simulink model "foc_pmsm"  (R2023a)
settings: Solver=VariableStepAuto  StartTime=0.0  StopTime=0.2  RelTol=1e-3
values from neighbouring files (symbols this model uses):
  L_d = 0.00113    [pmsm_init.m]    (also in pmsm_operating_points.m; pmsm_validation_compare.m)
  L_q = 0.00142    [pmsm_init.m]    (also in pmsm_operating_points.m; pmsm_validation_compare.m)
  polepairs = 3    [pmsm_init.m]    (also in pmsm_operating_points.m; pmsm_validation_compare.m)
  Psi_PM = 0.0169    [pmsm_init.m]    (also in pmsm_operating_points.m; pmsm_validation_compare.m)
  R_s = 0.543    [pmsm_init.m]    (also in pmsm_operating_points.m; pmsm_validation_compare.m)
  Ts = 1/10000    (= 0.0001)    [pmsm_init.m]    (also in pmsm_operating_points.m; pmsm_validation_compare.m)
  V_max = V_DC * max_modulation_index    [pmsm_init.m]    (also in pmsm_operating_points.m; pmsm_validation_compare.m)
undefined symbols (not defined in the file or in its folder): K_Id, K_Iq, K_Pd, K_Pq
libraries: slpidlib x2
settings Model: Creator=brogh  LastModifiedBy=hufnagelde
settings DataIOCC: SaveFormat=StructureWithTime
settings OptimizationCC: ReuseModelBlockBuffer=off
settings DebuggingCC: UnconnectedInputMsg=warning  UnconnectedOutputMsg=warning  UnconnectedLineMsg=warning
settings ModelReferenceCC: EnableRefExpFcnMdlSchedulingChecks=on
settings RTWCC: DLArmComputeVersion=19.05

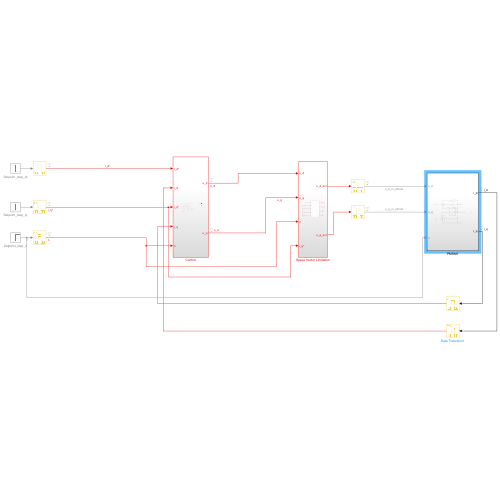
[thumbnail: Simulink's stored preview of the top-level diagram]
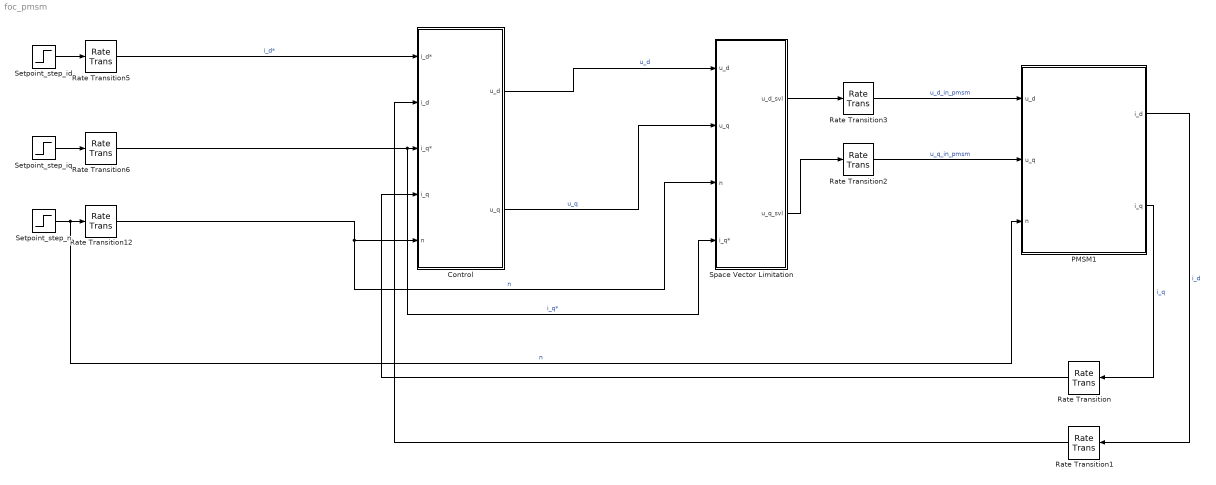
== system foc_pmsm ==
  Control : Subsystem
  PMSM1 : Subsystem
  Rate Transition{,1,5..6,12} (5 alike) : RateTransition  OutPortSampleTime=Ts
  Rate Transition2 : RateTransition  OutPortSampleTime=0
  Rate Transition3 : RateTransition  OutPortSampleTime=0
  Setpoint_step_id : Step  Time=0.1  After=-5  SampleTime=0
  Setpoint_step_iq : Step  Time=0.1  After=5  SampleTime=0
  Setpoint_step_n : Step  Time=0.03  Before=1000  After=1000  SampleTime=0
  Space Vector Limitation : Subsystem
  wires:
  Setpoint_step_id/1 -> Rate Transition5/1
  PMSM1/2(i_q) -> Rate Transition/1  "i_q"
  PMSM1/1(i_d) -> Rate Transition1/1  "i_d"
  Setpoint_step_iq/1 -> Rate Transition6/1
  Rate Transition/1 -> Control/4(i_q)
  Rate Transition1/1 -> Control/2(i_d)
  Rate Transition2/1 -> PMSM1/2(u_q)  "u_q_in_pmsm"
  Rate Transition3/1 -> PMSM1/1(u_d)  "u_d_in_pmsm"
  Rate Transition5/1 -> Control/1(i_d*)  "i_d*"
  Rate Transition6/1 -> Space Vector Limitation/4(i_q*), Control/3(i_q*)  "i_q*"
  Control/1(u_d) -> Space Vector Limitation/1(u_d)  "u_d"
  Control/2(u_q) -> Space Vector Limitation/2(u_q)  "u_q"
  Setpoint_step_n/1 -> Rate Transition12/1, PMSM1/3(n)  "n"
  Space Vector Limitation/1(u_d_svl) -> Rate Transition3/1
  Space Vector Limitation/2(u_q_svl) -> Rate Transition2/1
  Rate Transition12/1 -> Space Vector Limitation/3(n), Control/5(n)  "n"

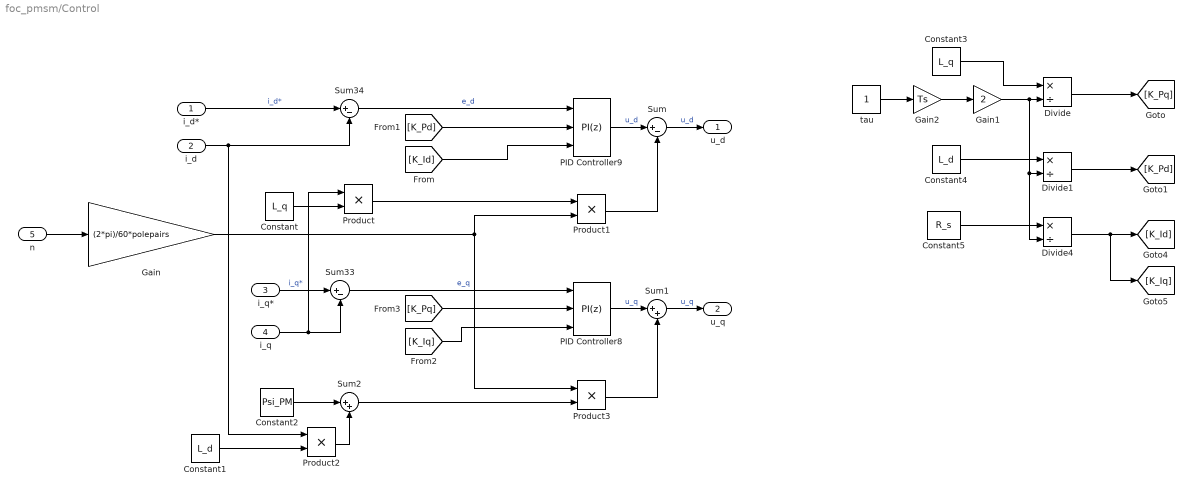
== system foc_pmsm/Control ==
  i_d* : Inport
  i_d : Inport  Port=2
  i_q* : Inport  Port=3
  i_q : Inport  Port=4
  n : Inport  Port=5
  Constant : Constant  Value=L_q
  Constant1 : Constant  Value=L_d
  Constant2 : Constant  Value=Psi_PM
  Constant3 : Constant  Value=L_q
  Constant4 : Constant  Value=L_d
  Constant5 : Constant  Value=R_s
  Divide : Product  Inputs=*/
  Divide1 : Product  Inputs=*/
  Divide4 : Product  Inputs=*/
  Gain : Gain  Gain=(2*pi)/60*polepairs
  Gain1 : Gain  Gain=2
  Gain2 : Gain  Gain=Ts
  PID Controller8 : slpidlib/PID Controller  Controller=PI  Form=Parallel  TimeDomain=Discrete-time  UseExternalTs=off  SampleTime=Ts  IntegratorMethod=Forward Euler  FilterMethod=Forward Euler  ControllerParametersSource=external  P=K_Pq  I=K_Iq  UseKiTs=off  D=0  N=100  UseFilter=on  TunerSelectOption=Transfer Function Based (PID Tuner App)  InitialConditionSource=internal  InitialConditionForIntegrator=0  InitialConditionForFilter=0  DifferentiatorICPrevScaledInput=0  ExternalReset=none  TrackingMode=off  Kt=1  LimitOutput=off  SatLimitsSource=internal  UpperSaturationLimit=36/sqrt(3)  LowerSaturationLimit=-36/sqrt(3)  LinearizeAsGain=on  AntiWindupMode=clamping  Kb=1  LimitIntegrator=off  UpperIntegratorSaturationLimit=inf  LowerIntegratorSaturationLimit=-inf  POutMin=[]  POutMax=[]  IOutMin=[]  IOutMax=[]  DOutMin=[]  DOutMax=[]  NOutMin=[]  NOutMax=[]  SumOutMin=[]  SumOutMax=[]  SaturationOutMin=[]  SaturationOutMax=[]  PParamMin=[]  PParamMax=[]  IParamMin=[]  IParamMax=[]  DParamMin=[]  DParamMax=[]  NParamMin=[]  NParamMax=[]  KbParamMin=[]  KbParamMax=[]  KtParamMin=[]  KtParamMax=[]  KbOutMin=[]  KbOutMax=[]  KtOutMin=[]  KtOutMax=[]  IntegratorOutMin=[]  IntegratorOutMax=[]  FilterOutMin=[]  FilterOutMax=[]  SumI1OutMin=[]  SumI1OutMax=[]  SumI2OutMin=[]  SumI2OutMax=[]  SumI3OutMin=[]  SumI3OutMax=[]  SumI4OutMin=[]  SumI4OutMax=[]  SumDOutMin=[]  SumDOutMax=[]  DifferentiatorOutMin=[]  DifferentiatorOutMax=[]  FilterDiffOutCoefMin=[]  FilterDiffOutCoefMax=[]  ReciprocalOutMin=[]  ReciprocalOutMax=[]  SumDenOutMin=[]  SumDenOutMax=[]  SumNumOutMin=[]  SumNumOutMax=[]  DivideOutMin=[]  DivideOutMax=[]  UdiffTsProdOutMin=[]  UdiffTsProdOutMax=[]  NTsProdOutMin=[]  NTsProdOutMax=[]  UintegralTsProdOutMin=[]  UintegralTsProdOutMax=[]  UngainTsProdOutMin=[]  UngainTsProdOutMax=[]  ClampingZeroOutDataTypeStr=Inherit: Inherit via back propagation  ClampingZeroOutMin=[]  ClampingZeroOutMax=[]  FilterDenConstantOutDataTypeStr=Inherit: Inherit via back propagation  FilterDenConstantOutMin=[]  FilterDenConstantOutMax=[]  PCopyOutDataTypeStr=Inherit: Inherit via back propagation  PCopyOutMin=[]  PCopyOutMax=[]  NCopyOutDataTypeStr=Inherit: Inherit via back propagation  NCopyOutMin=[]  NCopyOutMax=[]  IntegratorContinuousStateAttributes=''  IntegratorStateMustResolveToSignalObject=off  IntegratorRTWStateStorageClass=Auto  FilterContinuousStateAttributes=''  FilterStateMustResolveToSignalObject=off  FilterRTWStateStorageClass=Auto  ParallelPVariant=ExternalParameters  IdealPVariant=Disabled  IVariant=ExternalParameters  DVariant=Disabled  IntegratorVariant=Discrete  SatVariant=Disabled  AWVariant=Passthrough  PCopyVariant=Disabled  TRVariant=Disabled  FdbkBlocksVariant=Forward  IdealPFdbkVariant=Disabled  SatFdbkVariant=Disabled  DerivativeFilterVariant=Disabled  NVariant=Disabled  NCopyVariant=Disabled_SignalSpec  FilterICVariant=Disabled  IntegratorICVariant=InternalICs  ExternalResetVariant=Disabled  TRSumVariant=Passthrough  SumFdbkVariant=Disabled  SumVariant=Sum_PI  TsampFilterVariant=InternalTs  TsampNgainVariant=Passthrough  TsampIntegralVariant=Disabled_SignalSpec  ExternalSaturationOutDataTypeStr=Inherit: Same as second input
  PID Controller9 : slpidlib/PID Controller  Controller=PI  Form=Parallel  TimeDomain=Discrete-time  UseExternalTs=off  SampleTime=Ts  IntegratorMethod=Forward Euler  FilterMethod=Forward Euler  ControllerParametersSource=external  P=K_Pd  I=K_Id  UseKiTs=off  D=0  N=100  UseFilter=on  TunerSelectOption=Transfer Function Based (PID Tuner App)  InitialConditionSource=internal  InitialConditionForIntegrator=0  InitialConditionForFilter=0  DifferentiatorICPrevScaledInput=0  ExternalReset=none  TrackingMode=off  Kt=1  LimitOutput=off  SatLimitsSource=internal  UpperSaturationLimit=36/sqrt(3)  LowerSaturationLimit=-36/sqrt(3)  LinearizeAsGain=on  AntiWindupMode=none  Kb=1  LimitIntegrator=off  UpperIntegratorSaturationLimit=inf  LowerIntegratorSaturationLimit=-inf  POutMin=[]  POutMax=[]  IOutMin=[]  IOutMax=[]  DOutMin=[]  DOutMax=[]  NOutMin=[]  NOutMax=[]  SumOutMin=[]  SumOutMax=[]  SaturationOutMin=[]  SaturationOutMax=[]  PParamMin=[]  PParamMax=[]  IParamMin=[]  IParamMax=[]  DParamMin=[]  DParamMax=[]  NParamMin=[]  NParamMax=[]  KbParamMin=[]  KbParamMax=[]  KtParamMin=[]  KtParamMax=[]  KbOutMin=[]  KbOutMax=[]  KtOutMin=[]  KtOutMax=[]  IntegratorOutMin=[]  IntegratorOutMax=[]  FilterOutMin=[]  FilterOutMax=[]  SumI1OutMin=[]  SumI1OutMax=[]  SumI2OutMin=[]  SumI2OutMax=[]  SumI3OutMin=[]  SumI3OutMax=[]  SumI4OutMin=[]  SumI4OutMax=[]  SumDOutMin=[]  SumDOutMax=[]  DifferentiatorOutMin=[]  DifferentiatorOutMax=[]  FilterDiffOutCoefMin=[]  FilterDiffOutCoefMax=[]  ReciprocalOutMin=[]  ReciprocalOutMax=[]  SumDenOutMin=[]  SumDenOutMax=[]  SumNumOutMin=[]  SumNumOutMax=[]  DivideOutMin=[]  DivideOutMax=[]  UdiffTsProdOutMin=[]  UdiffTsProdOutMax=[]  NTsProdOutMin=[]  NTsProdOutMax=[]  UintegralTsProdOutMin=[]  UintegralTsProdOutMax=[]  UngainTsProdOutMin=[]  UngainTsProdOutMax=[]  ClampingZeroOutDataTypeStr=Inherit: Inherit via back propagation  ClampingZeroOutMin=[]  ClampingZeroOutMax=[]  FilterDenConstantOutDataTypeStr=Inherit: Inherit via back propagation  FilterDenConstantOutMin=[]  FilterDenConstantOutMax=[]  PCopyOutDataTypeStr=Inherit: Inherit via back propagation  PCopyOutMin=[]  PCopyOutMax=[]  NCopyOutDataTypeStr=Inherit: Inherit via back propagation  NCopyOutMin=[]  NCopyOutMax=[]  IntegratorContinuousStateAttributes=''  IntegratorStateMustResolveToSignalObject=off  IntegratorRTWStateStorageClass=Auto  FilterContinuousStateAttributes=''  FilterStateMustResolveToSignalObject=off  FilterRTWStateStorageClass=Auto  ParallelPVariant=ExternalParameters  IdealPVariant=Disabled  IVariant=ExternalParameters  DVariant=Disabled  IntegratorVariant=Discrete  SatVariant=Disabled  AWVariant=Passthrough  PCopyVariant=Disabled  TRVariant=Disabled  FdbkBlocksVariant=Forward  IdealPFdbkVariant=Disabled  SatFdbkVariant=Disabled  DerivativeFilterVariant=Disabled  NVariant=Disabled  NCopyVariant=Disabled_SignalSpec  FilterICVariant=Disabled  IntegratorICVariant=InternalICs  ExternalResetVariant=Disabled  TRSumVariant=Passthrough  SumFdbkVariant=Disabled  SumVariant=Sum_PI  TsampFilterVariant=InternalTs  TsampNgainVariant=Passthrough  TsampIntegralVariant=Disabled_SignalSpec  ExternalSaturationOutDataTypeStr=Inherit: Same as second input
  Product{,1..3} (4 alike) : Product
  Sum : Sum  Inputs=|+-
  Sum1 : Sum  Inputs=|++
  Sum2 : Sum  Inputs=|++
  Sum33 : Sum  Inputs=|+-
  Sum34 : Sum  Inputs=|+-
  tau : Constant
  u_d : Outport
  u_q : Outport  Port=2
  wires:
  PID Controller9/1 -> Sum/1  "u_d"
  Divide1/1 -> [K_Pd]
  Product/1 -> Product1/1
  Constant4/1 -> Divide1/1
  tau/1 -> Gain2/1
  Sum/1 -> u_d/1  "u_d"
  Divide4/1 -> [K_Iq], [K_Id]
  [K_Iq] -> PID Controller8/3
  Divide/1 -> [K_Pq]
  [K_Id] -> PID Controller9/3
  Constant5/1 -> Divide4/1
  Product2/1 -> Sum2/2
  n/1 -> Gain/1
  [K_Pd] -> PID Controller9/2
  Gain1/1 -> Divide4/2, Divide1/2, Divide/2
  Constant2/1 -> Sum2/1
  i_d/1 -> Sum34/2, Product2/1
  Sum33/1 -> PID Controller8/1  "e_q"
  Constant1/1 -> Product2/2
  i_q/1 -> Sum33/2, Product/1
  i_d*/1 -> Sum34/1  "i_d*"
  i_q*/1 -> Sum33/1  "i_q*"
  Sum34/1 -> PID Controller9/1  "e_d"
  PID Controller8/1 -> Sum1/1  "u_q"
  Sum1/1 -> u_q/1  "u_q"
  Constant3/1 -> Divide/1
  Sum2/1 -> Product3/2
  Constant/1 -> Product/2
  [K_Pq] -> PID Controller8/2
  Gain2/1 -> Gain1/1
  Gain/1 -> Product3/1, Product1/2
  Product3/1 -> Sum1/2
  Product1/1 -> Sum/2

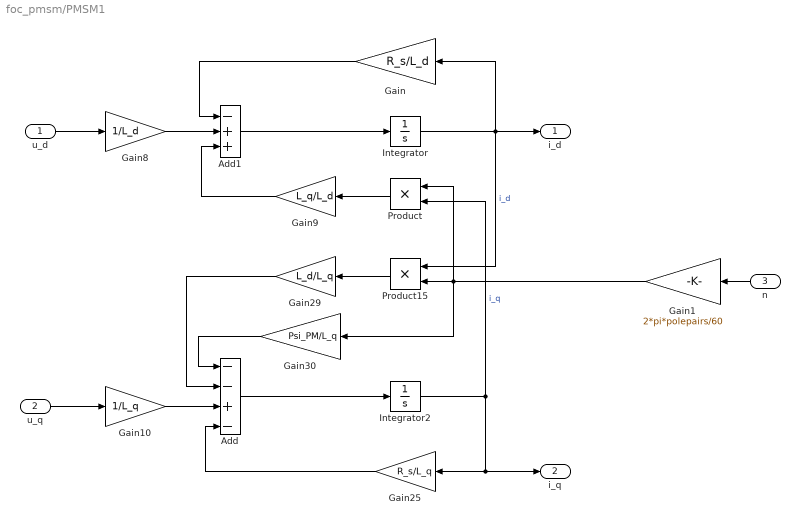
== system foc_pmsm/PMSM1 ==
  u_d : Inport
  u_q : Inport  Port=2
  n : Inport  Port=3
  Add : Sum  Inputs=--+-
  Add1 : Sum  Inputs=-++
  Gain : Gain  Gain=R_s/L_d
  Gain1 : Gain  Gain=2*pi*polepairs/60
  Gain10 : Gain  Gain=1/L_q
  Gain25 : Gain  Gain=R_s/L_q
  Gain29 : Gain  Gain=L_d/L_q
  Gain30 : Gain  Gain=Psi_PM/L_q
  Gain8 : Gain  Gain=1/L_d
  Gain9 : Gain  Gain=L_q/L_d
  Integrator : Integrator
  Integrator2 : Integrator
  Product : Product
  Product15 : Product
  i_d : Outport
  i_q : Outport  Port=2
  wires:
  n/1 -> Gain1/1
  u_d/1 -> Gain8/1
  Integrator/1 -> i_d/1, Product15/1, Gain/1  "i_d"
  Gain25/1 -> Add/4
  Product15/1 -> Gain29/1
  Add1/1 -> Integrator/1
  Add/1 -> Integrator2/1
  Gain9/1 -> Add1/3
  Gain8/1 -> Add1/2
  Gain10/1 -> Add/3
  Gain/1 -> Add1/1
  u_q/1 -> Gain10/1
  Product/1 -> Gain9/1
  Gain29/1 -> Add/2
  Integrator2/1 -> i_q/1, Gain25/1, Product/2  "i_q"
  Gain30/1 -> Add/1
  Gain1/1 -> Gain30/1, Product/1, Product15/2

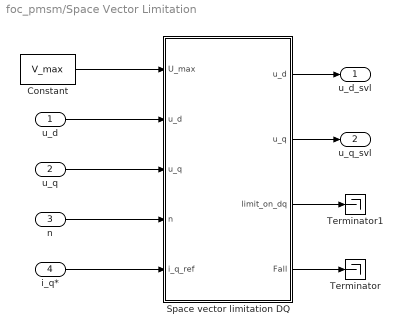
== system foc_pmsm/Space Vector Limitation ==
  u_d : Inport
  u_q : Inport  Port=2
  n : Inport  Port=3
  i_q* : Inport  Port=4
  Constant : Constant  Value=V_max
  Space vector limitation DQ : MATLAB Function  TreatAsAtomicUnit=on
  Terminator : Terminator
  Terminator1 : Terminator
  u_d_svl : Outport
  u_q_svl : Outport  Port=2
  wires:
  u_d/1 -> Space vector limitation DQ/2("u_d ")
  u_q/1 -> Space vector limitation DQ/3("u_q ")
  n/1 -> Space vector limitation DQ/4(n)
  Space vector limitation DQ/1(u_d) -> u_d_svl/1
  Constant/1 -> Space vector limitation DQ/1(U_max)
  Space vector limitation DQ/3(limit_on_dq) -> Terminator1/1
  i_q*/1 -> Space vector limitation DQ/5(i_q_ref)
  Space vector limitation DQ/2(u_q) -> u_q_svl/1
  Space vector limitation DQ/4(Fall) -> Terminator/1

== matlab function foc_pmsm/Space Vector Limitation/Space vector limitation DQ ==
  data: U_max input; u_d input; u_d output; u_q input; u_q output; n input; i_q_ref input; limit_on_dq output; Fall output
function [u_d, u_q, limit_on_dq, Fall] = fcn(U_max, u_d, u_q, n, i_q_ref)

U_abs = sqrt(u_d^2 + u_q^2); % tatsächlicher Betrag des Spannungsraumzeigers
U_max_SF = U_max;
% Ist eine Begrenzung notwendig?
if ( U_abs > U_max_SF )
    limit_on_dq = boolean(1);
    
    % Motor- oder Generatorbetrieb?
    if ((sign(n))==(sign(i_q_ref))) % Motorbetrieb

        if (abs(u_d) > (0.95*U_max_SF))
            u_d_lim = sign(u_d) * 0.95 * U_max_SF;
            u_q_lim = sign(u_q) * sqrt(U_max_SF^2 - u_d_lim^2);
            Fall=1;
        else
            u_d_lim = u_d;
            u_q_lim = sign(u_q) * sqrt(U_max_SF^2 - u_d_lim^2);
            Fall=2;
        end
    

    else % Generatorbetrieb
        
        if ((abs(u_q)) > (0.95*U_max_SF))
            u_q_lim = sign(u_q) * 0.95 * U_max_SF;
            u_d_lim = sign(u_d) * sqrt(U_max_SF^2 - u_q_lim^2);
            Fall=3;
        else
            u_q_lim = u_q;
            u_d_lim = sign(u_d) * sqrt(U_max_SF^2 - u_q_lim^2);
            Fall=4;
        end

    end    

else % keine Begrenzung nötig
    u_d_lim = u_d;
    u_q_lim = u_q;
    limit_on_dq = boolean(0);
    Fall=5;
end

u_d = u_d_lim;
u_q = u_q_lim;

end
